simulink model "threephase_SVPWM"  (R2015a)
settings: Solver=ode45  StartTime=0.0  StopTime=0.1  MaxStep=0.00001  MinStep=0.000001  RelTol=1e-3
libraries: powerlib x31, simulink x1
settings Model: Creator=hp  LastModifiedBy=hp
settings SolverCC: ZeroCrossControl=DisableAll

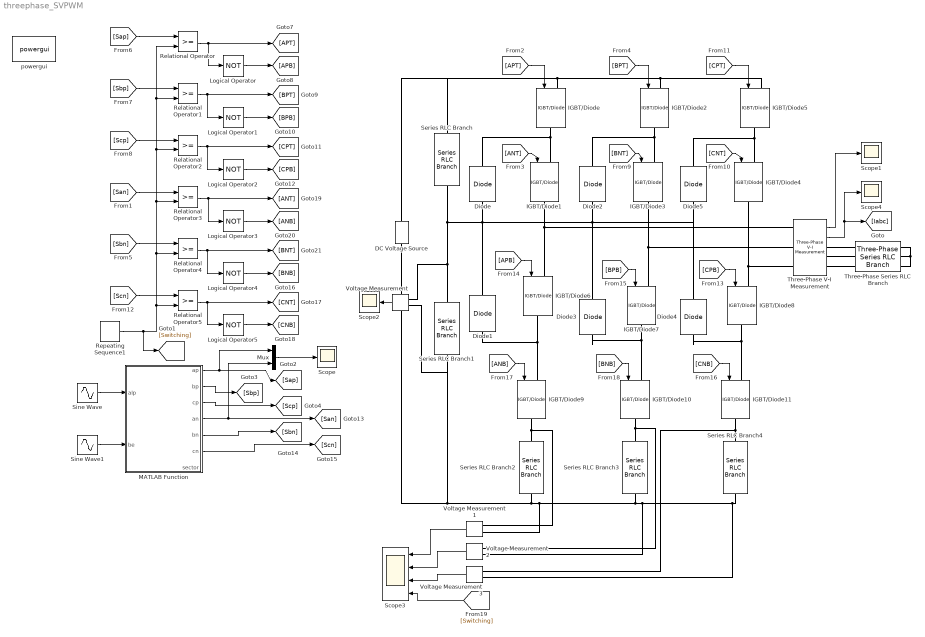
== system threephase_SVPWM ==
  DC Voltage Source : powerlib/Electrical Sources/DC Voltage Source  Amplitude=400  Measurements=None
  Diode{,1..5} (6 alike) : powerlib/Power Electronics/Diode  Ron=0.001  Lon=0  Vf=0.8  IC=0  UseSnubber=off  Rs=500  Cs=250e-9  Measurements=off
  IGBT/Diode{,1..11} (12 alike) : powerlib/Power Electronics/IGBT//Diode  Ron=1e-3  Rs=1e5  Cs=inf  Measurements=off
  Logical Operator{,1..5} (6 alike) : Logic  Operator=NOT  Inputs=1  AllPortsSameDT=off  OutDataTypeStr=boolean
  MATLAB Function : MATLAB Function  TreatAsAtomicUnit=on
  Mux : Mux  Inputs=2
  Relational Operator{,1..5} (6 alike) : RelationalOperator  OutDataTypeStr=boolean
  Repeating Sequence1 : simulink/Sources/Repeating Sequence  rep_seq_t=[0 0.5 1]/1000  rep_seq_y=[0 1 0]
  Scope{,1..2,4} (4 alike) : Scope
      Scope1 settings: YMin=-400  YMax=400
      Scope2 settings: YMin=-10  YMax=210  SaveName=ScopeData2
      Scope4 settings: YMin=-22.5  YMax=20  SaveName=ScopeData5
  Scope3 : Scope  NumInputPorts=4
      settings: YMin=-10~-5~-5~-5  YMax=210~5~5~5  SaveName=ScopeData3
  Series RLC Branch : powerlib/Elements/Series RLC Branch  LConnTagsString=__new0  RConnTagsString=__new0  BranchType=RC  Resistance=0.1  Inductance=1e-3  SetiL0=off  InitialCurrent=0  Capacitance=7700e-6  Setx0=off  InitialVoltage=0  Measurements=None
  Series RLC Branch1 : powerlib/Elements/Series RLC Branch  LConnTagsString=__new0  RConnTagsString=__new0  BranchType=RC  Resistance=0.1  Inductance=1e-3  SetiL0=off  InitialCurrent=0  Capacitance=7700e-6  Setx0=off  InitialVoltage=0  Measurements=None
  Series RLC Branch2 : powerlib/Elements/Series RLC Branch  LConnTagsString=__new0  RConnTagsString=__new0  BranchType=R  Resistance=0.001  Inductance=1e-3  SetiL0=off  InitialCurrent=0  Capacitance=1e-6  Setx0=off  InitialVoltage=0  Measurements=None
  Series RLC Branch3 : powerlib/Elements/Series RLC Branch  LConnTagsString=__new0  RConnTagsString=__new0  BranchType=R  Resistance=0.001  Inductance=1e-3  SetiL0=off  InitialCurrent=0  Capacitance=1e-6  Setx0=off  InitialVoltage=0  Measurements=None
  Series RLC Branch4 : powerlib/Elements/Series RLC Branch  LConnTagsString=__new0  RConnTagsString=__new0  BranchType=R  Resistance=0.001  Inductance=1e-3  SetiL0=off  InitialCurrent=0  Capacitance=1e-6  Setx0=off  InitialVoltage=0  Measurements=None
  Sine Wave : Sin  Frequency=2*pi*50  SampleTime=0
  Sine Wave1 : Sin  Frequency=2*pi*50  Phase=pi/2  SampleTime=0
  Three-Phase Series RLC Branch : powerlib/Elements/Three-Phase Series RLC Branch  LConnTagsString=A|B|C  RConnTagsString=A|B|C  BranchType=RLC  Resistance=10  Inductance=10e-3  Capacitance=0  Measurements=None
  Three-Phase V-I Measurement : powerlib/Measurements/Three-Phase V-I Measurement  VoltageMeasurement=phase-to-phase  SetLabelV=off  LabelV=Vabc  Vpu=off  VpuLL=off  CurrentMeasurement=yes  SetLabelI=off  LabelI=Iabc  Ipu=off  Pbase=100e6  Vbase=500e3  OutputType=Complex  PhasorSimulation=off  PSBequivalent=0
  Voltage Measurement{,1..3} (4 alike) : powerlib/Measurements/Voltage Measurement  PhasorSimulation=off  OutputType=Complex  PSBequivalent=0
  powergui : powerlib/powergui  Priority=1  SimulationMode=Continuous  SolverType=Tustin/Backward Euler (TBE)  SampleTime=2e-6  frequency=60  SPID=off  DisableSnubberDevices=off  DisableRonSwitches=off  DisableVfSwitches=off  SwTol=0  DisplayEquations=off  Interpol=off  methode=off  Ts=100  FunctionMessages=off  echomessages=off  HookPort=off  EnableUseOfTLC=off  x0status=blocks  frequencyindice=0  Pbase=100e6  ErrMax=1e-4  Iterations=50  UnitsV=kV  UnitsW=MW  buscounter=0  RestoreLinks=warning  ResistiveCurrentMeasurement=off  Frange=[0:2:500]  Ylog=off  Xlog=on  ShowGrid=off  save=off  variable=ZData  structure=0  ZoomFFT=off  StartTime=0.0  cycles=1  DisplayStyle=1  fundamental=60  FreqAxis=off  MaxFrequency=1000  frequencyindicesteady=1  RmsSteady=1  display=off
  wires:
  MATLAB Function/1(ap) -> Mux/1, [Sap]
  MATLAB Function/2(bp) -> [Sbp]
  MATLAB Function/3(cp) -> [Scp]
  Three-Phase V-I Measurement/2 -> Scope4/1, [Iabc]
  Sine Wave/1 -> MATLAB Function/1(alp)
  Sine Wave1/1 -> MATLAB Function/2(be)
  [Sap] -> Relational Operator/1
  [Sbp] -> Relational Operator1/1
  [Scp] -> Relational Operator2/1
  Relational Operator/1 -> Logical Operator/1, [APT]
  Logical Operator/1 -> [APB]
  Relational Operator1/1 -> Logical Operator1/1, [BPT]
  Logical Operator1/1 -> [BPB]
  Relational Operator2/1 -> Logical Operator2/1, [CPT]
  Logical Operator2/1 -> [CPB]
  [APT] -> IGBT/Diode/1
  [ANT] -> IGBT/Diode1/1
  [BPT] -> IGBT/Diode2/1
  [BNT] -> IGBT/Diode3/1
  [CNT] -> IGBT/Diode4/1
  [CPT] -> IGBT/Diode5/1
  MATLAB Function/4(an) -> [San], Mux/2
  MATLAB Function/5(bn) -> [Sbn]
  MATLAB Function/6(cn) -> [Scn]
  [San] -> Relational Operator3/1
  Repeating Sequence1/1 -> [Switching], Relational Operator5/2, Relational Operator4/2, Relational Operator3/2, Relational Operator2/2, Relational Operator/2, Relational Operator1/2
  [Sbn] -> Relational Operator4/1
  [Scn] -> Relational Operator5/1
  Relational Operator3/1 -> Logical Operator3/1, [ANT]
  Logical Operator3/1 -> [ANB]
  Relational Operator4/1 -> Logical Operator4/1, [BNT]
  Logical Operator4/1 -> [BNB]
  Relational Operator5/1 -> Logical Operator5/1, [CNT]
  Logical Operator5/1 -> [CNB]
  [APB] -> IGBT/Diode6/1
  [BPB] -> IGBT/Diode7/1
  [CPB] -> IGBT/Diode8/1
  [ANB] -> IGBT/Diode9/1
  [BNB] -> IGBT/Diode10/1
  [CNB] -> IGBT/Diode11/1
  Three-Phase V-I Measurement/1 -> Scope1/1
  Mux/1 -> Scope/1
  Voltage Measurement/1 -> Scope2/1
  [Switching] -> Scope3/4
  Voltage Measurement3/1 -> Scope3/3
  Voltage Measurement2/1 -> Scope3/2
  Voltage Measurement1/1 -> Scope3/1
  connections:
  Three-Phase Series RLC Branch/RConn1 -- Three-Phase Series RLC Branch/RConn2 -- Three-Phase Series RLC Branch/RConn3
  Three-Phase V-I Measurement/RConn1 -- Three-Phase Series RLC Branch/LConn1
  Three-Phase V-I Measurement/RConn2 -- Three-Phase Series RLC Branch/LConn2
  Three-Phase V-I Measurement/RConn3 -- Three-Phase Series RLC Branch/LConn3
  IGBT/Diode/RConn1 -- Diode/RConn1 -- IGBT/Diode1/LConn1
  IGBT/Diode2/RConn1 -- Diode2/RConn1 -- IGBT/Diode3/LConn1
  IGBT/Diode5/RConn1 -- Diode5/RConn1 -- IGBT/Diode4/LConn1
  IGBT/Diode/LConn1 -- Series RLC Branch/LConn1 -- DC Voltage Source/RConn1 -- IGBT/Diode2/LConn1 -- IGBT/Diode5/LConn1
  IGBT/Diode7/RConn1 -- Diode3/LConn1 -- IGBT/Diode10/LConn1
  IGBT/Diode8/RConn1 -- IGBT/Diode11/LConn1 -- Diode4/LConn1
  IGBT/Diode6/RConn1 -- Diode1/LConn1 -- IGBT/Diode9/LConn1
  IGBT/Diode3/RConn1 -- IGBT/Diode7/LConn1 -- Three-Phase V-I Measurement/LConn2
  IGBT/Diode6/LConn1 -- Three-Phase V-I Measurement/LConn1 -- IGBT/Diode1/RConn1
  Series RLC Branch1/LConn1 -- Voltage Measurement/LConn1 -- Diode5/LConn1 -- Diode4/RConn1 -- Diode2/LConn1 -- Diode3/RConn1 -- Diode/LConn1 -- Diode1/RConn1 -- Series RLC Branch/RConn1
  IGBT/Diode8/LConn1 -- IGBT/Diode4/RConn1 -- Three-Phase V-I Measurement/LConn3
  Series RLC Branch4/RConn1 -- Voltage Measurement3/LConn2 -- Voltage Measurement2/LConn2 -- Series RLC Branch3/RConn1 -- Voltage Measurement1/LConn2 -- Series RLC Branch2/RConn1 -- Voltage Measurement/LConn2 -- Series RLC Branch1/RConn1 -- DC Voltage Source/LConn1
  Series RLC Branch2/LConn1 -- Voltage Measurement1/LConn1 -- IGBT/Diode9/RConn1
  Series RLC Branch3/LConn1 -- Voltage Measurement2/LConn1 -- IGBT/Diode10/RConn1
  Series RLC Branch4/LConn1 -- Voltage Measurement3/LConn1 -- IGBT/Diode11/RConn1

== matlab function threephase_SVPWM/MATLAB Function ==
  data: alp input; ap output; be input; bp output; cp output; an output; bn output; cn output; sector output
function [ap,bp,cp,an,bn,cn,sector] = fcn(alp,be)
%#codegen
	sec_a=0,sec_b=0,sec_c=0;
	t_o = 0,ta = 0,tb = 0,tc = 0,tsec = 0;

    sec_a = be;										%Beta;
	sec_b = ((-be/2)+(alp*0.866));			%(-0.5*Beta+(0.866*alpha));
	sec_c = ((-be/2)-(alp*0.866));			%(-0.5*Beta-(0.866*alpha));
    
    if(sec_a>=0)
       if(sec_b>=0)
       												%	sector 1
    		t_o = (1 - (sec_a+sec_b))/2;							%	t_1 = sec_b, t_2 =sec_a
    		ta = sec_a+sec_b+(t_o);
    		tb  = sec_a+(t_o);
    		tc  = (t_o);
            tsec = 1;
       else
            if(sec_c>=0)												%	sector 3
        		t_o = (1 - (sec_a+sec_c))/2;						%	t_1 = sec_a, t_2 =sec_c
        		ta = (t_o);
        		tb = sec_a+sec_c+(t_o);
        		tc = sec_c+(t_o);
                tsec = 3;
            else												%	sector 2
        		t_o = (1 + (sec_c+sec_b))/2;					%	t_1 = -sec_c, t_2 =-sec_b
        		ta = -sec_c+(t_o);
        		tb = -(sec_c+sec_b)+(t_o);
        		tc = (t_o);
                tsec = 2;
            end
       end
    else
       if(sec_b>=0)
           if(sec_c>=0)                                                  %	sector 5
        		t_o = (1 - (sec_c+sec_b))/2; 				%	t_1 = sec_c, t_2 =sec_b
        		ta = sec_b+(t_o);
        		tb = (t_o);
        		tc = sec_c+sec_b+(t_o);
                tsec = 5;
           else                                                  %	sector 6
        		t_o = (1 + (sec_a+sec_c))/2; 				%	t_1 = -sec_a, t_2 =-sec_c
        		ta = -(sec_a+sec_c)+(t_o);
        		tb = (t_o);
        		tc = -sec_a+(t_o);
                tsec = 6;
           end
       else
            if(sec_c>=0)                                      %	sector 4
        		t_o = (1 + (sec_a+sec_b))/2;			%	t_1 = -sec_b, t_2 =-sec_a
        		ta = (t_o);
        		tb = -sec_b+(t_o);
        		tc = -(sec_a+sec_b)+(t_o);
                tsec = 4;
            end
       end
    end

if(ta>0.5)
    ap = (2*ta)-1;
    an = 1;
else
    ap = 0;
    an = 2*ta;
end

if(tb>0.5)
    bp = (2*tb)-1;
    bn = 1;
else
    bp = 0;
    bn = 2*tb;
end

if(tc>0.5)
    cp = (2*tc)-1;
    cn = 1;
else
    cp = 0;
    cn = 2*tc;
end

sector = tsec;
